simulink model "cart_pendulum"  (R2018b)
settings: Solver=ode45  StartTime=0.0  StopTime=5  MaxStep=0.005  RelTol=1e-8  AbsTol=1e-10
model workspace (MAT data in the model file):
  I = 0.006
  M = 0.5
  b = 0.1
  force_ts = [0  0; 5  0]
  g = 9.8
  l = 0.3
  m = 0.2
  z0 = [0; 0; 0.0872664625997; 0]
settings Model: Creator=volka  LastModifiedBy=volka
settings DataIOCC: ReturnWorkspaceOutputs=on

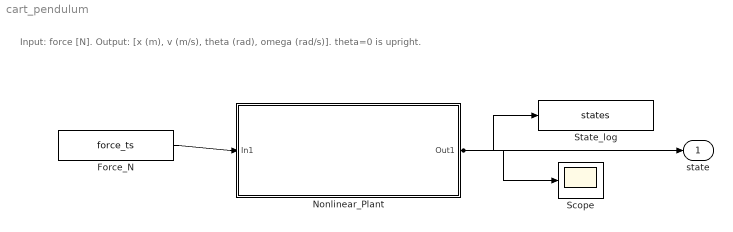
== system cart_pendulum ==
  note: Input: force [N]. Output: [x (m), v (m/s), theta (rad), omega (rad/s)]. theta=0 is upright.
  Force_N : FromWorkspace  VariableName=force_ts  SampleTime=0  Interpolate=off  OutputAfterFinalValue=Holding final value
  Nonlinear_Plant : Subsystem
  Scope : Scope
  State_log : ToWorkspace  VariableName=states  SaveFormat=Structure With Time  SampleTime=-1
  state : Outport
  wires:
  Force_N/1 -> Nonlinear_Plant/1(In1)
  Nonlinear_Plant/1(Out1) -> State_log/1, Scope/1, state/1

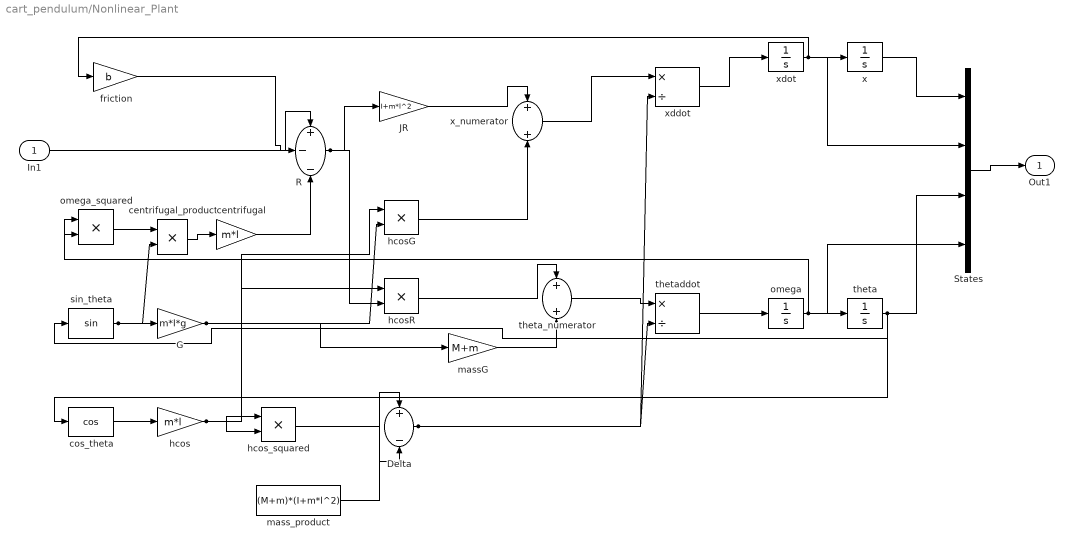
== system cart_pendulum/Nonlinear_Plant ==
  In1 : Inport
  Delta : Sum  Inputs=+-
  G : Gain  Gain=m*l*g
  JR : Gain  Gain=I+m*l^2
  R : Sum  Inputs=+--
  States : Mux
  centrifugal : Gain  Gain=m*l
  centrifugal_product : Product  Inputs=**
  cos_theta : Trigonometry  Operator=cos
  friction : Gain  Gain=b
  hcos : Gain  Gain=m*l
  hcosG : Product  Inputs=**
  hcosR : Product  Inputs=**
  hcos_squared : Product  Inputs=**
  massG : Gain  Gain=M+m
  mass_product : Constant  Value=(M+m)*(I+m*l^2)
  omega : Integrator  InitialCondition=z0(4)
  omega_squared : Product  Inputs=**
  sin_theta : Trigonometry
  theta : Integrator  InitialCondition=z0(3)
  theta_numerator : Sum
  thetaddot : Product  Inputs=*/
  x : Integrator  InitialCondition=z0(1)
  x_numerator : Sum
  xddot : Product  Inputs=*/
  xdot : Integrator  InitialCondition=z0(2)
  Out1 : Outport
  wires:
  In1/1 -> R/1
  xdot/1 -> friction/1, x/1, States/2
  friction/1 -> R/2
  omega/1 -> omega_squared/1, omega_squared/2, theta/1, States/4
  omega_squared/1 -> centrifugal_product/1
  theta/1 -> sin_theta/1, cos_theta/1, States/3
  sin_theta/1 -> centrifugal_product/2, G/1
  centrifugal_product/1 -> centrifugal/1
  centrifugal/1 -> R/3
  cos_theta/1 -> hcos/1
  hcos/1 -> hcos_squared/1, hcos_squared/2, hcosG/1, hcosR/1
  mass_product/1 -> Delta/1
  hcos_squared/1 -> Delta/2
  R/1 -> JR/1, hcosR/2
  G/1 -> hcosG/2, massG/1
  JR/1 -> x_numerator/1
  hcosG/1 -> x_numerator/2
  hcosR/1 -> theta_numerator/1
  massG/1 -> theta_numerator/2
  x_numerator/1 -> xddot/1
  Delta/1 -> xddot/2, thetaddot/2
  theta_numerator/1 -> thetaddot/1
  xddot/1 -> xdot/1
  thetaddot/1 -> omega/1
  x/1 -> States/1
  States/1 -> Out1/1
